simulink model "PMSGRectifiedBlockWindEq"  (R2021b)
settings: Solver=VariableStepAuto  StartTime=0.0  StopTime=20  RelTol=1e-7
values from neighbouring files (symbols this model uses):
  breakpoints1 = cp_data(2:end,1)'    [FullCodePMSGData.m]
  breakpoints2 = cp_data(1,2:end)    [FullCodePMSGData.m]
  RL = 20    [ForMotorCricuitREpesentationRectifiedDiodes.m]    (also in FullCodePMSGData.m = 117.2980678)
  RPM_Wind_table_data = cp_data(2:end,2:end)    [FullCodePMSGData.m]
  Windspeed = 14    [ForMotorCricuitREpesentationRectifiedDiodes.m]    (also in FullCodePMSGData.m = 11)
libraries: spsSeriesRLCBranchLib x5, spsVoltageMeasurementLib x3, spsCurrentMeasurementLib x1, spsPermanentMagnetSynchronousMachineLib x1, spsUniversalBridgeLib x1, spspowerguiLib x1
settings Model: Creator=glopezc  LastModifiedBy=cheog
settings DebuggingCC: UnconnectedInputMsg=none  UnconnectedOutputMsg=none  UnconnectedLineMsg=none
settings RTWCC: DLArmComputeVersion=20.02.1

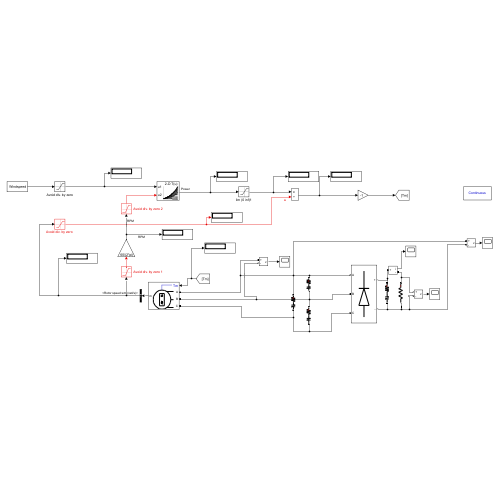
[thumbnail: Simulink's stored preview of the top-level diagram]
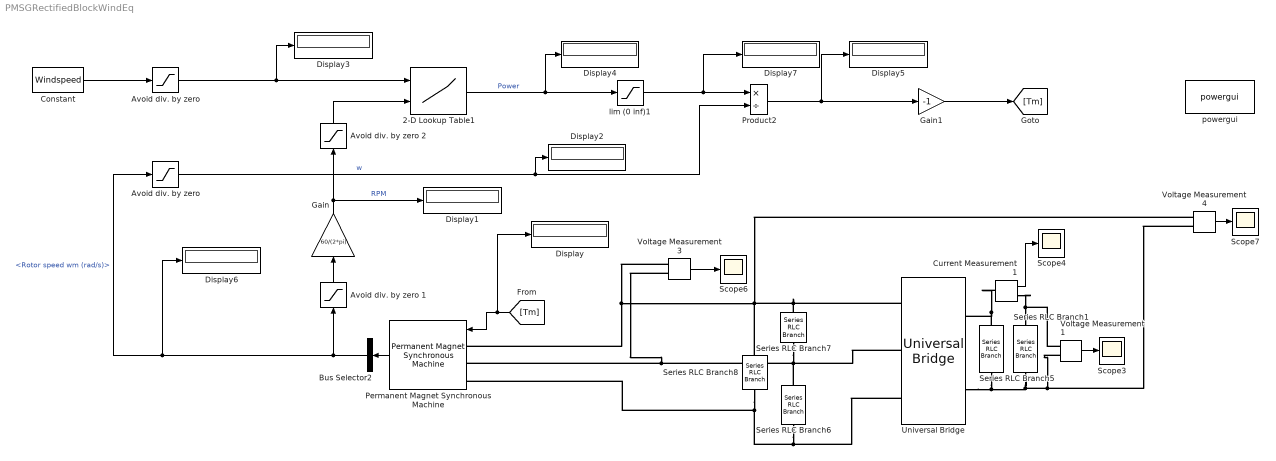
== system PMSGRectifiedBlockWindEq ==
  2-D Lookup Table1 : Lookup_n-D  BreakpointsForDimension1=breakpoints1  BreakpointsForDimension2=breakpoints2  BreakpointsForDimension1DataTypeStr=double  BreakpointsForDimension2DataTypeStr=double  Table=RPM_Wind_table_data  InternalRulePriority=Speed  OutDataTypeStr=double  RndMeth=Simplest  InputSameDT=on
      settings: InputPortMap=u0,u1
  Avoid div. by zero : Saturate  UpperLimit=inf  LowerLimit=eps
  "Avoid div. by zero " : Saturate  UpperLimit=inf  LowerLimit=eps
  Avoid div. by zero 1 : Saturate  UpperLimit=inf  LowerLimit=eps
  Avoid div. by zero 2 : Saturate  UpperLimit=inf  LowerLimit=eps
  Bus Selector2 : BusSelector  OutputSignals=Rotor speed wm (rad/s)
  Constant : Constant  Value=Windspeed
  Current Measurement1 : spsCurrentMeasurementLib/Current Measurement  PhasorSimulation=off  OutputType=Complex  PSBequivalent=0
  Display{,1..7} (8 alike) : Display
  Gain : Gain  Gain=60/(2*pi)
  Gain1 : Gain  Gain=-1
  Permanent Magnet Synchronous Machine : spsPermanentMagnetSynchronousMachineLib/Permanent Magnet Synchronous Machine  NbPhases=3  FluxDistribution=Sinusoidal  RotorType=Salient-pole  MechanicalLoad=Torque Tm  PresetModel=No  ShowDetailedParameters=on  MeasurementBus=off  Resistance=0.51  Inductance=8.5e-3  dqInductances=[0.0128 0.0128]  La=0.0128  MachineConstant=Voltage Constant (V_peak L-L / krpm)  Flux=3.3941  VoltageCst=9850.0043  TorqueCst=81.4589  Flat=120  Mechanical=[175 0 16 5]  PolePairs=4  InitialConditions=[0,0, 0,0]  InitialConditions5ph=[0 0 0 0 0 0]  RefAngle=90 degrees behind phase A axis (modified Park)  IterativeDiscreteModel=Trapezoidal non iterative  TsBlock=-1  TsPowergui=0
  Product2 : Product  Inputs=*/  InputSameDT=on  SaturateOnIntegerOverflow=on  OutDataTypeStr=Inherit: Same as first input
  Scope{3..4,6..7} (4 alike) : Scope
  Series RLC Branch1 : spsSeriesRLCBranchLib/Series RLC Branch  LConnTagsString=__new0  RConnTagsString=__new0  BranchType=R  Resistance=RL  Inductance=1e-3  SetiL0=off  InitialCurrent=0  Capacitance=1e-6  Setx0=off  InitialVoltage=0  Measurements=None
  Series RLC Branch5 : spsSeriesRLCBranchLib/Series RLC Branch  LConnTagsString=__new0  RConnTagsString=__new0  BranchType=RC  Resistance=.00084  Inductance=1e-3  SetiL0=off  InitialCurrent=0  Capacitance=2200e-6  Setx0=off  InitialVoltage=0  Measurements=None
  Series RLC Branch6 : spsSeriesRLCBranchLib/Series RLC Branch  LConnTagsString=__new0  RConnTagsString=__new0  BranchType=RC  Resistance=0.001  Inductance=1e-3  SetiL0=off  InitialCurrent=0  Capacitance=55e-6  Setx0=off  InitialVoltage=0  Measurements=None
  Series RLC Branch7 : spsSeriesRLCBranchLib/Series RLC Branch  LConnTagsString=__new0  RConnTagsString=__new0  BranchType=RC  Resistance=0.001  Inductance=1e-3  SetiL0=off  InitialCurrent=0  Capacitance=55e-6  Setx0=off  InitialVoltage=0  Measurements=None
  Series RLC Branch8 : spsSeriesRLCBranchLib/Series RLC Branch  LConnTagsString=__new0  RConnTagsString=__new0  BranchType=RC  Resistance=0.001  Inductance=1e-3  SetiL0=off  InitialCurrent=0  Capacitance=55e-6  Setx0=off  InitialVoltage=0  Measurements=None
  Universal Bridge : spsUniversalBridgeLib/Universal Bridge  Arms=3  SnubberResistance=Rd  SnubberCapacitance=Cd  Device=Diodes  Ron=1e-2  Lon=0  ForwardVoltages="[  0  0  ]"  ForwardVoltage=0.6  GTOparameters=[ 10e-6 , 20e-6 ]  IGBTparameters=[ 1e-6 , 2e-6 ]  Measurements=None  Measurements_2=None  converterType=Rectifier
  Voltage Measurement1 : spsVoltageMeasurementLib/Voltage Measurement  PhasorSimulation=off  OutputType=Complex  PSBequivalent=0
  Voltage Measurement3 : spsVoltageMeasurementLib/Voltage Measurement  PhasorSimulation=off  OutputType=Complex  PSBequivalent=0
  Voltage Measurement4 : spsVoltageMeasurementLib/Voltage Measurement  PhasorSimulation=off  OutputType=Complex  PSBequivalent=0
  lim (0 inf)1 : Saturate  UpperLimit=inf  LowerLimit=eps
  powergui : spspowerguiLib/powergui  Priority=1  SimulationMode=Continuous  SampleTime=50e-6  frequency=60  Iterations=50  frequencyindice=0  Pbase=100e6  ErrMax=1e-4  UnitsV=kV  UnitsW=MW  buscounter=0  FunctionMessages=off  echomessages=off  EnableUseOfTLC=off  CurrentSourceSwitches=off  DisableSnubberDevices=off  DisableRonSwitches=off  DisableVfSwitches=off  DisplayEquations=off  AutomaticDiscreteSolvers=off  SolverType=Tustin/Backward Euler (TBE)  Interpol=off  ExternalGateDelay=off  methode=off  Ts=100  x0status=blocks  SPID=on  SwTol=0  HookPort=off  NonlinearTolerance=1e-4  nMaxIteration=100  ContinueOnMaxIteration=off  RestoreLinks=warning  ResistiveCurrentMeasurement=off  Frange=[0:2:500]  Ylog=off  Xlog=on  ShowGrid=off  save=off  variable=ZData  structure=0  ZoomFFT=off  StartTime=0.0  cycles=1  DisplayStyle=1  fundamental=60  FreqAxis=off  MaxFrequency=1000  frequencyindicesteady=1  RmsSteady=1  display=off
  wires:
  Current Measurement1/1 -> Scope4/1
  Voltage Measurement1/1 -> Scope3/1
  Voltage Measurement3/1 -> Scope6/1
  Voltage Measurement4/1 -> Scope7/1
  lim (0 inf)1/1 -> Display7/1, Product2/1
  Constant/1 -> Avoid div. by zero/1
  2-D Lookup Table1/1 -> Display4/1, lim (0 inf)1/1  "Power"
  Bus Selector2/1 -> Display6/1, "Avoid div. by zero "/1, Avoid div. by zero 1/1  "<Rotor speed wm (rad/s)>"
  Avoid div. by zero/1 -> Display3/1, 2-D Lookup Table1/1
  Gain/1 -> Display1/1, Avoid div. by zero 2/1  "RPM"
  [Tm] -> Display/1, Permanent Magnet Synchronous Machine/1
  Permanent Magnet Synchronous Machine/1 -> Bus Selector2/1
  Avoid div. by zero 1/1 -> Gain/1
  "Avoid div. by zero "/1 -> Product2/2, Display2/1  "w"
  Product2/1 -> Gain1/1, Display5/1
  Gain1/1 -> [Tm]
  Avoid div. by zero 2/1 -> 2-D Lookup Table1/2
  connections:
  Series RLC Branch6/RConn1 -- Universal Bridge/LConn3 -- Series RLC Branch8/RConn1 -- Permanent Magnet Synchronous Machine/LConn3
  Series RLC Branch7/RConn1 -- Universal Bridge/LConn2 -- Series RLC Branch6/LConn1 -- Voltage Measurement3/LConn2 -- Permanent Magnet Synchronous Machine/LConn2
  Permanent Magnet Synchronous Machine/LConn1 -- Voltage Measurement3/LConn1 -- Universal Bridge/LConn1 -- Series RLC Branch7/LConn1 -- Voltage Measurement4/LConn1 -- Series RLC Branch8/LConn1
  Voltage Measurement4/LConn2 -- Voltage Measurement1/LConn2 -- Series RLC Branch5/RConn1 -- Universal Bridge/RConn2 -- Series RLC Branch1/RConn1
  Current Measurement1/RConn1 -- Voltage Measurement1/LConn1 -- Series RLC Branch1/LConn1
  Series RLC Branch5/LConn1 -- Universal Bridge/RConn1 -- Current Measurement1/LConn1
